simulink model "syncGenInfBusNoIfSimulink"  (R2013a)
settings: Solver=ode4  StartTime=0.0  StopTime=10.0  FixedStep=0.001  RelTol=1e-3
undefined symbols (not defined in the file): D_p, delta0, i_d0, i_f, i_q0, J, L_s, m, omega0, omega_g, R_s, T_m, V
settings Model: Creator=USER  LastModifiedBy=USER

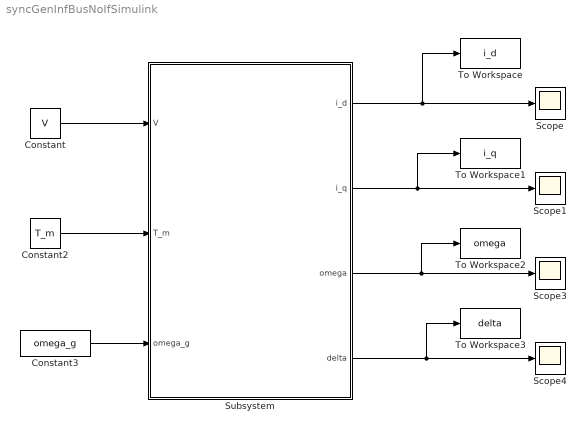
== system syncGenInfBusNoIfSimulink ==
  Constant : Constant  Value=V
  Constant2 : Constant  Value=T_m
  Constant3 : Constant  Value=omega_g
  Scope{,1,3..4} (4 alike) : Scope
      Scope3 settings: TimeRange=10  YMin=300  YMax=900  SaveName=ScopeData3
      Scope4 settings: SaveName=ScopeData4
  Subsystem : Subsystem
  To Workspace : ToWorkspace  VariableName=i_d  SampleTime=-1  SaveFormat=Timeseries
  To Workspace1 : ToWorkspace  VariableName=i_q  SampleTime=-1  SaveFormat=Timeseries
  To Workspace2 : ToWorkspace  VariableName=omega  SampleTime=-1  SaveFormat=Timeseries
  To Workspace3 : ToWorkspace  VariableName=delta  SampleTime=-1  SaveFormat=Timeseries
  wires:
  Subsystem/1(i_d) -> To Workspace/1, Scope/1
  Subsystem/2("i_q ") -> To Workspace1/1, Scope1/1
  Subsystem/4(delta) -> To Workspace3/1, Scope4/1
  Constant/1 -> Subsystem/1(V)
  Constant2/1 -> Subsystem/2(T_m)
  Constant3/1 -> Subsystem/3(omega_g)
  Subsystem/3(omega) -> To Workspace2/1, Scope3/1

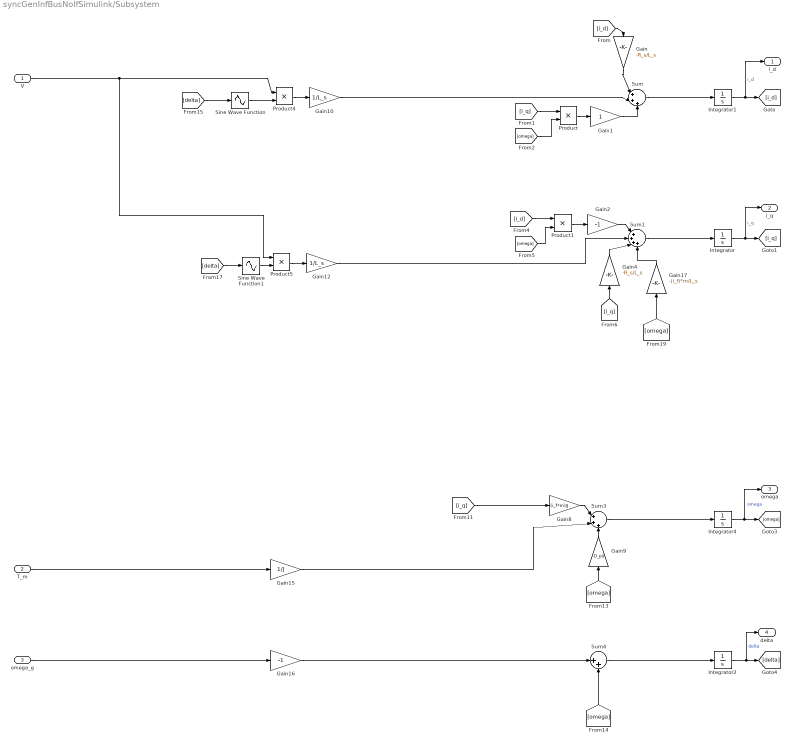
== system syncGenInfBusNoIfSimulink/Subsystem ==
  V : Inport
  T_m : Inport  Port=2
  omega_g : Inport  Port=3
  Gain : Gain  Gain=-R_s/L_s
  Gain1 : Gain
  Gain10 : Gain  Gain=1/L_s
  Gain12 : Gain  Gain=1/L_s
  Gain15 : Gain  Gain=1/J
  Gain16 : Gain  Gain=-1
  Gain17 : Gain  Gain=-(i_f)*m/L_s
  Gain2 : Gain  Gain=-1
  Gain4 : Gain  Gain=-R_s/L_s
  Gain8 : Gain  Gain=(i_f*m)/J
  Gain9 : Gain  Gain=-D_p/J
  Integrator : Integrator  InitialCondition=i_q0
  Integrator1 : Integrator  InitialCondition=i_d0
  Integrator2 : Integrator  InitialCondition=delta0
  Integrator4 : Integrator  InitialCondition=omega0
  Product{,1,4..5} (4 alike) : Product
  Sine Wave Function : Sin  TimeSource=Use external signal  SampleTime=0
  Sine Wave Function1 : Sin  TimeSource=Use external signal  Phase=pi/2  SampleTime=0
  Sum : Sum  Inputs=|+++
  Sum1 : Sum  Inputs=|++++
  Sum3 : Sum  Inputs=|+++
  Sum4 : Sum  Inputs=|++
  i_d : Outport
  "i_q " : Outport  Port=2
  omega : Outport  Port=3
  delta : Outport  Port=4
  wires:
  Integrator1/1 -> i_d/1, [i_d]  "i_d"
  Integrator/1 -> "i_q "/1, [i_q]  "i_q"
  Integrator4/1 -> omega/1, [omega]  "omega"
  Integrator2/1 -> delta/1, [delta]  "delta"
  Sum/1 -> Integrator1/1
  [i_d] -> Gain/1
  Gain/1 -> Sum/1
  Product/1 -> Gain1/1
  [i_q] -> Product/1
  [omega] -> Product/2
  Gain1/1 -> Sum/3
  Sum1/1 -> Integrator/1
  Gain2/1 -> Sum1/1
  Product1/1 -> Gain2/1
  [i_d] -> Product1/1
  [omega] -> Product1/2
  Gain4/1 -> Sum1/3
  [i_q] -> Gain4/1
  Sum3/1 -> Integrator4/1
  Gain8/1 -> Sum3/1
  Gain9/1 -> Sum3/3
  [omega] -> Gain9/1
  [i_q] -> Gain8/1
  Sum4/1 -> Integrator2/1
  [omega] -> Sum4/2
  Gain10/1 -> Sum/2
  Sine Wave Function/1 -> Product4/2
  [delta] -> Sine Wave Function/1
  Product4/1 -> Gain10/1
  Gain12/1 -> Sum1/2
  Sine Wave Function1/1 -> Product5/2
  [delta] -> Sine Wave Function1/1
  Product5/1 -> Gain12/1
  V/1 -> Product5/1, Product4/1
  T_m/1 -> Gain15/1
  Gain15/1 -> Sum3/2
  omega_g/1 -> Gain16/1
  Gain16/1 -> Sum4/1
  [omega] -> Gain17/1
  Gain17/1 -> Sum1/4
